simulink model "example1"  (Simulink 7.9)
settings: Solver=ode45  StartTime=0.0  StopTime=10.0  RelTol=1e-3
settings Model: Creator=CAST  LastModifiedBy=CAST

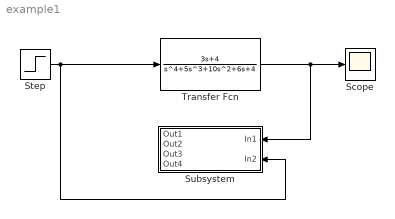
== system example1 ==
  Scope : Scope
  Step : Step  Time=0  After=10  SampleTime=0.05
  Subsystem : Subsystem  RequirementInfo="{}  %GIDa_28fe6724_fa33_499b_aac5_f38d22268b2d"
  Transfer Fcn : TransferFcn  Numerator=[3 4]  Denominator=[1 5 10 6 4]
  wires:
  Step/1 -> Transfer Fcn/1, Subsystem/2(In2)
  Transfer Fcn/1 -> Scope/1, Subsystem/1(In1)

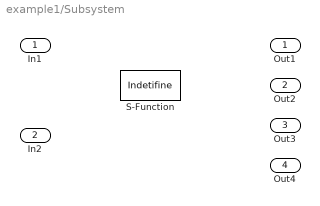
== system example1/Subsystem ==
  In1 : Inport
  In2 : Inport  Port=2
  S-Function : S-Function  FunctionName=Indetifine  EnableBusSupport=off
  Out1 : Outport
  Out2 : Outport  Port=2
  Out3 : Outport  Port=3
  Out4 : Outport  Port=4
